simulink model "pv_and_wind_completed"  (R2018a)
settings: Solver=VariableStepAuto  StartTime=0.0  StopTime=2.4  RelTol=1e-3
libraries: powerlib x50, powerlib_meascontrol x12, simulink x10, re_lib x2, peGeneralControl x1, simulink_extras x1
(part 2 of 2)

== matlab function pv_and_wind_completed/Active Power Filter/MATLAB Function1 ==
  data: Valpha input; Ialpha_ref output; Vbeta input; p_ref input; q_ref input; Ibeta_ref output
function [Ialpha_ref, Ibeta_ref] = calc_I_alphabeta(Valpha, Vbeta, p_ref, q_ref)
% CALC_I_ALPHABETA Calculates reference currents in the alpha-beta frame
% 
% Inputs:
%   Valpha    - Instantaneous alpha-voltage
%   Vbeta     - Instantaneous beta-voltage
%   p_ref     - Active power reference (p*)
%   q_ref     - Reactive power reference (q*)
%
% Outputs:
%   Ialpha_ref - Reference current in alpha-axis
%   Ibeta_ref  - Reference current in beta-axis

    % Calculate the voltage magnitude squared
    v_sq = Valpha^2 + Vbeta^2;
    
    % Avoid division by zero when supply voltage drops to zero
    if v_sq < 1e-6
        v_sq = 1e-6;
    end

    % Matrix transformation equations:
    % [Ialpha_ref] = (1 / (Valpha^2 + Vbeta^2)) * [ Valpha  -Vbeta ] * [ p_ref ]
    % [Ibeta_ref ]                               [ Vbeta    Valpha ]   [ q_ref ]

    Ialpha_ref = (1 / v_sq) * (Valpha * p_ref - Vbeta * q_ref);
    Ibeta_ref  = (1 / v_sq) * (Vbeta * p_ref + Valpha * q_ref);
    
end
